simulink model "Neurofeedback_Errorfunction"  (R2022a)
settings: Solver=FixedStepAuto  StartTime=0.0  StopTime=300  FixedStep=1  RelTol=1e-3
libraries: simulink x2
settings Model: Creator=mariodelossantos  LastModifiedBy=mariodelossantos

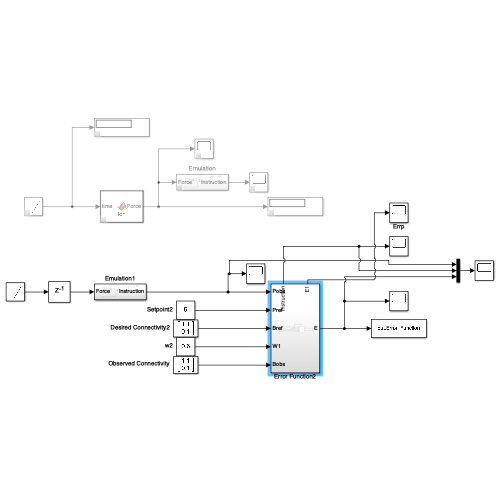
[thumbnail: Simulink's stored preview of the top-level diagram]
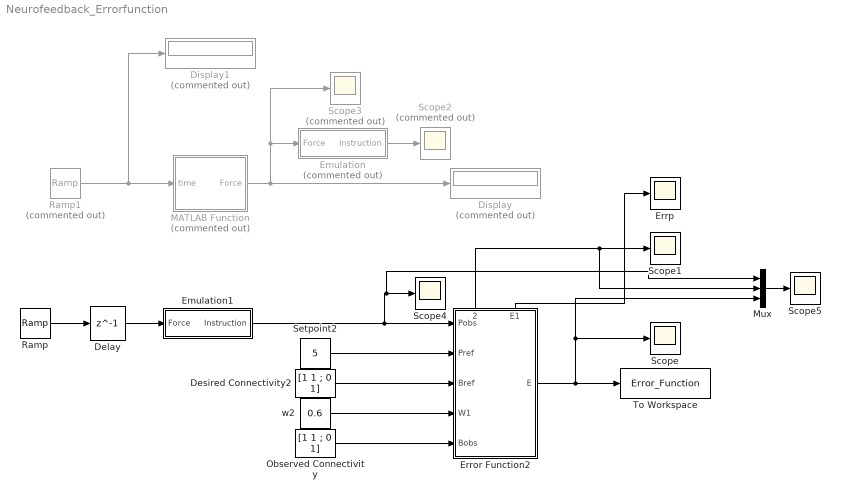
== system Neurofeedback_Errorfunction ==
  Delay : Delay  DelayLength=1  InitialCondition=0
  Desired Connectivity2 : Constant  Value="[1   1 ; 0  1]"
  Display : Display  Commented=on
  Display1 : Display  Commented=on
  Emulation : Subsystem  Commented=on
  Emulation1 : Subsystem
  Error Function2 : Subsystem
      settings: PortSchema="{\"entries\":[{\"content\":{\"sides\":[{\"content\":{\"connectorIds\":[\"In1\",\"In2\",\"In3\",\"In4\",\"In5\"]},\"type\":\"ConnectorPlacement.EquallySpacedRectSide\",\"uuid\":\"444fbf9f-83f0-405e-b780-73f2a519e5d8\"},{\"content\":{\"connectorIds\":[\"Out1\"],\"side\":\"RIGHT\"},\"type\":\"ConnectorPlacement.EquallySpacedRectSide\",\"uuid\":\"580feeb9-eb76-4e38-ada2-7c0fba9b3602\"},{\"content\":{\"connectorIds\":[\"Out2\",\"Out3\"],\"side\":\"TOP\"},\"type\":\"ConnectorPlacement.EquallySpacedRectSide\",\"uuid\":\"86f5bef5-f023-4b75-b93f-dc016b73225e\"}]},\"type\":\"ConnectorPlacement.EquallySpacedConnector\",\"uuid\":\"50bb9fda-b7f3-427b-ab4c-df885dc392aa\"}],\"packageUris\":[\"http://schema.mathworks.com/mf0/Connector/R2020b\"],\"version\":\"1.0\"}"
  Errp : Scope
  MATLAB Function : MATLAB Function  Commented=on  TreatAsAtomicUnit=on
  Mux : Mux  Inputs=3
  Observed Connectivity : Constant  Value="[1   1 ; 0  1]"
  Ramp : simulink/Sources/Ramp  slope=0.03  start=0  InitialOutput=1
  Ramp1 : simulink/Sources/Ramp  Commented=on  slope=0.1  start=0  InitialOutput=0
  Scope{,1,4..5} (4 alike) : Scope
  Scope2 : Scope  Commented=on
  Scope3 : Scope  Commented=on
  Setpoint2 : Constant  Value=5
  To Workspace : ToWorkspace  VariableName=Error_Function  SaveFormat=Timeseries  SampleTime=-1
  w2 : Constant  Value=0.6
  wires:
  w2/1 -> Error Function2/4(W1)
  Setpoint2/1 -> Error Function2/2(Pref)
  Desired Connectivity2/1 -> Error Function2/3(Bref)
  Observed Connectivity/1 -> Error Function2/5(Bobs)
  Error Function2/1(E) -> Mux/3, Scope/1, To Workspace/1
  Error Function2/2(Instruction) -> Mux/2, Scope1/1
  Ramp1/1 -> Display1/1, MATLAB Function/1(time)
  Emulation/1(Instruction) -> Scope2/1
  MATLAB Function/1(Force) -> Display/1, Emulation/1(Force), Scope3/1
  Ramp/1 -> Delay/1
  Emulation1/1(Instruction) -> Mux/1, Scope4/1, Error Function2/1(Pobs)
  Delay/1 -> Emulation1/1(Force)
  Mux/1 -> Scope5/1
  Error Function2/3(E1) -> Errp/1

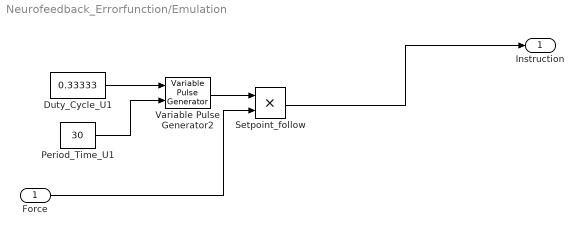
== system Neurofeedback_Errorfunction/Emulation ==
  Force : Inport
  Duty_Cycle_U1 : Constant  Value=0.33333  OutMin=[0]  OutMax=[0.8]
  Period_Time_U1 : Constant  Value=30
  Setpoint_follow : Product
  Variable Pulse Generator2 : VariablePulseGenerator  AllowZeroPulseWidth=on  RunAtFixedTimeIntervals=on
  Instruction : Outport
  wires:
  Setpoint_follow/1 -> Instruction/1
  Duty_Cycle_U1/1 -> Variable Pulse Generator2/1
  Variable Pulse Generator2/1 -> Setpoint_follow/1
  Force/1 -> Setpoint_follow/2
  Period_Time_U1/1 -> Variable Pulse Generator2/2

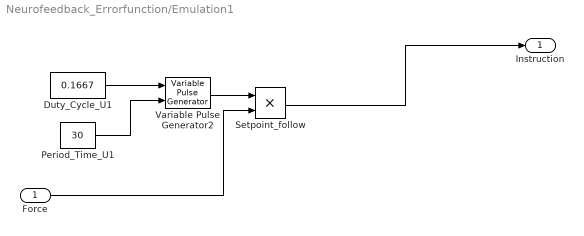
== system Neurofeedback_Errorfunction/Emulation1 ==
  Force : Inport
  Duty_Cycle_U1 : Constant  Value=0.1667  OutMin=[0]  OutMax=[0.8]
  Period_Time_U1 : Constant  Value=30
  Setpoint_follow : Product
  Variable Pulse Generator2 : VariablePulseGenerator  AllowZeroPulseWidth=on  RunAtFixedTimeIntervals=on
  Instruction : Outport
  wires:
  Setpoint_follow/1 -> Instruction/1
  Duty_Cycle_U1/1 -> Variable Pulse Generator2/1
  Variable Pulse Generator2/1 -> Setpoint_follow/1
  Force/1 -> Setpoint_follow/2
  Period_Time_U1/1 -> Variable Pulse Generator2/2

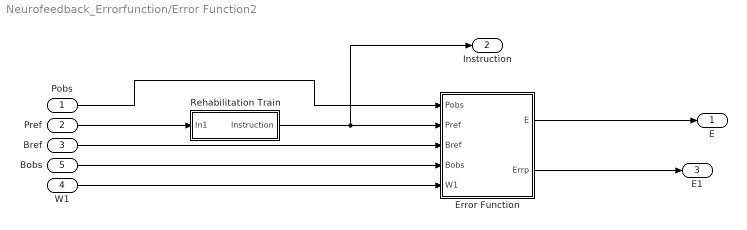
== system Neurofeedback_Errorfunction/Error Function2 ==
  Pobs : Inport
  Pref : Inport  Port=2
  Bref : Inport  Port=3
  W1 : Inport  Port=4
  Bobs : Inport  Port=5
  Error Function : Subsystem
  Rehabilitation Train : Subsystem
  E : Outport
  Instruction : Outport  Port=2
  E1 : Outport  Port=3
  wires:
  Bref/1 -> Error Function/3(Bref)
  Bobs/1 -> Error Function/4(Bobs)
  W1/1 -> Error Function/5(W1)
  Pref/1 -> Rehabilitation Train/1(In1)
  Pobs/1 -> Error Function/1(Pobs)
  Rehabilitation Train/1(Instruction) -> Instruction/1, Error Function/2(Pref)
  Error Function/1(E) -> E/1
  Error Function/2(Errp) -> E1/1

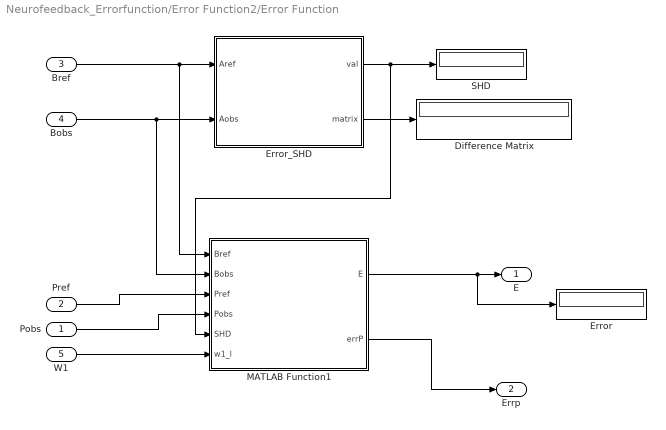
== system Neurofeedback_Errorfunction/Error Function2/Error Function ==
  Pobs : Inport
  Pref : Inport  Port=2
  Bref : Inport  Port=3
  Bobs : Inport  Port=4
  W1 : Inport  Port=5
  Difference Matrix : Display
  Error : Display
  Error_SHD : MATLAB Function  TreatAsAtomicUnit=on
  MATLAB Function1 : MATLAB Function  TreatAsAtomicUnit=on
  SHD : Display
  E : Outport
  Errp : Outport  Port=2
  wires:
  Error_SHD/2(matrix) -> Difference Matrix/1
  Bref/1 -> MATLAB Function1/1(Bref), Error_SHD/1(Aref)
  Error_SHD/1(val) -> MATLAB Function1/5(SHD), SHD/1
  Bobs/1 -> MATLAB Function1/2(Bobs), Error_SHD/2(Aobs)
  Pobs/1 -> MATLAB Function1/4(Pobs)
  Pref/1 -> MATLAB Function1/3(Pref)
  W1/1 -> MATLAB Function1/6(w1_l)
  MATLAB Function1/1(E) -> Error/1, E/1
  MATLAB Function1/2(errP) -> Errp/1

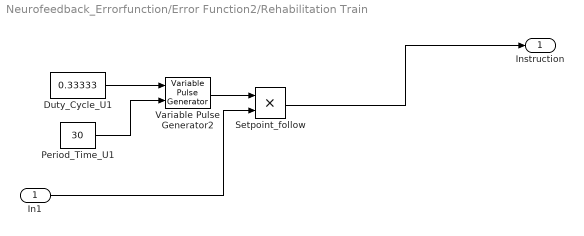
== system Neurofeedback_Errorfunction/Error Function2/Rehabilitation Train ==
  In1 : Inport
  Duty_Cycle_U1 : Constant  Value=0.33333  OutMin=[0]  OutMax=[0.8]
  Period_Time_U1 : Constant  Value=30
  Setpoint_follow : Product
  Variable Pulse Generator2 : VariablePulseGenerator  AllowZeroPulseWidth=on  RunAtFixedTimeIntervals=on
  Instruction : Outport
  wires:
  Setpoint_follow/1 -> Instruction/1
  Duty_Cycle_U1/1 -> Variable Pulse Generator2/1
  Variable Pulse Generator2/1 -> Setpoint_follow/1
  In1/1 -> Setpoint_follow/2
  Period_Time_U1/1 -> Variable Pulse Generator2/2

== matlab function Neurofeedback_Errorfunction/MATLAB Function ==
  data: Force output; time input
function Force  = fcn(time)

%Function to increase force each determined time, we are not considering
%the actual error

I = 0:30:300; % Tiempo de cambio
temp = 0;
for i = 1:10
    if time == I(i)
        temp = time / I(i);
    end
end

Force = temp;

== matlab function Neurofeedback_Errorfunction/Error Function2/Error Function/Error_SHD ==
  data: Aref input; val output; Aobs input; matrix output
function [val,matrix]=SHD(Aref,Aobs)

val = sum(sum(xor(Aref,Aobs)));
matrix = xor(Aref,Aobs);

== matlab function Neurofeedback_Errorfunction/Error Function2/Error Function/MATLAB Function1 ==
  data: Bref input; E output size=1; Bobs input; Pref input; Pobs input; SHD input; w1_l input; errP output
function [E,errP]  = ErrorFunction(Bref, Bobs, Pref, Pobs, SHD, w1_l)
    w1 = w1_l; %Use whatever values you like most. Threshold 

    w2 = 1 - w1;

    assert(all(size(Bref) == size(Bobs)));

    assert(size(Bref,1) == size(Bref,2));

    nChannels = size(Bref,1);

    BfullyConnected = ones(nChannels);

    BfullyDisconnected = zeros(nChannels);

   
    maxDiffSHD= sum(sum(xor(BfullyConnected,BfullyDisconnected))); %SHD
    errA = SHD/maxDiffSHD; %Normalize error in the connectivity
    %errP = (abs(Pref-Pobs))/abs(Pref);

    errP = exp(-1/(Pobs-Pref) + eps);
    
E = (w1 * errA + w2 * errP);
